simulink model "SimulinkLabPartOne"  (R2024b)
settings: Solver=VariableStepAuto  StartTime=0.0  StopTime=10.0  RelTol=1e-3
libraries: simulink x6
settings Model: Creator=ferbe  LastModifiedBy=ferbe

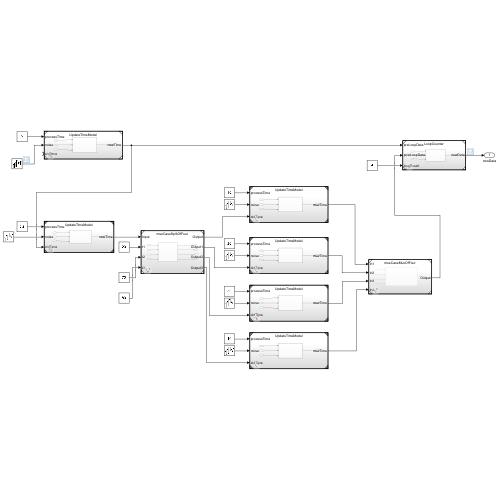
[thumbnail: Simulink's stored preview of the top-level diagram]
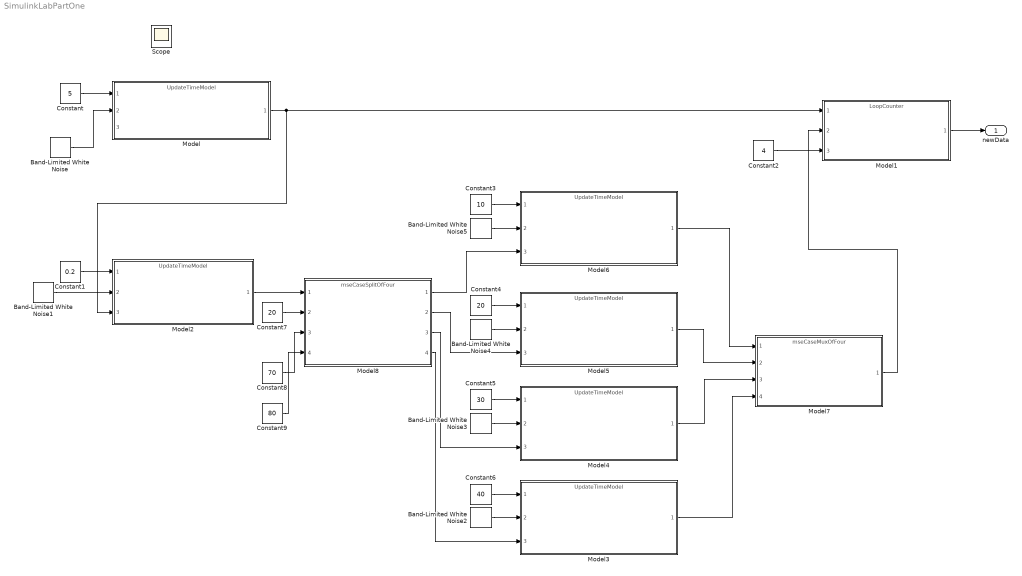
== system SimulinkLabPartOne ==
  Band-Limited White Noise{,1..5} (6 alike) : simulink/Sources/Band-Limited White Noise  Cov=[0.1]  Ts=0.1  seed=[23341]
  Constant : Constant  Value=5
  Constant1 : Constant  Value=0.2
  Constant2 : Constant  Value=4
  Constant3 : Constant  Value=10
  Constant4 : Constant  Value=20
  Constant5 : Constant  Value=30
  Constant6 : Constant  Value=40
  Constant7 : Constant  Value=20
  Constant8 : Constant  Value=70
  Constant9 : Constant  Value=80
  Model{,2..6} (6 alike) : ModelReference  ModelNameDialog=UpdateTimeModel.slx  SimulationMode=Normal  ModelReferenceVersion=5.2
  Model1 : ModelReference  ModelNameDialog=LoopCounter.slx  SimulationMode=Normal  ModelReferenceVersion=5.0
  Model7 : ModelReference  ModelNameDialog=mseCaseMuxOfFour.slx  SimulationMode=Normal  ModelReferenceVersion=1.5
  Model8 : ModelReference  ModelNameDialog=mseCaseSplitOfFour.slx  SimulationMode=Normal  ModelReferenceVersion=1.13
  newData : Outport
  Scope : Scope
  wires:
  Band-Limited White Noise/1 -> Model/2
  Constant/1 -> Model/1
  Constant2/1 -> Model1/3
  Constant1/1 -> Model2/1
  Band-Limited White Noise1/1 -> Model2/2
  Model/1 -> Model2/3, Model1/1
  Band-Limited White Noise5/1 -> Model6/2
  Band-Limited White Noise4/1 -> Model5/2
  Band-Limited White Noise3/1 -> Model4/2
  Band-Limited White Noise2/1 -> Model3/2
  Constant3/1 -> Model6/1
  Constant4/1 -> Model5/1
  Constant5/1 -> Model4/1
  Constant6/1 -> Model3/1
  Model6/1 -> Model7/1
  Model5/1 -> Model7/2
  Model3/1 -> Model7/4
  Model7/1 -> Model1/2
  Model4/1 -> Model7/3
  Model2/1 -> Model8/1
  Model8/1 -> Model6/3
  Model8/2 -> Model5/3
  Model8/3 -> Model4/3
  Model8/4 -> Model3/3
  Model1/1 -> newData/1
  Constant7/1 -> Model8/2
  Constant8/1 -> Model8/3
  Constant9/1 -> Model8/4
